simulink model "Model_6DOF"  (R2020b)
settings: Solver=FixedStepAuto  StartTime=0.0  StopTime=Tfin  FixedStep=0.05  RelTol=1e-3
values from neighbouring files (symbols this model uses):
  Ba_0 = [0 0 0 0 0 0]    [ctrl_mode_param.m]
  Bb = 4418825.3321    [load_data.m]
  Bv_0 = [tgt_speed 0 0 0 0 0]    [ctrl_mode_param.m]
  Bx_0 = [0 0 tgt_depth 0 0 0]    [ctrl_mode_param.m]
  check_angle = 10    [ctrl_mode_param.m]
  ctrl_mode = 2    [run.m]
  dX_imposed = 10    [ctrl_mode_param.m]
  Ixx = 5.23e7    (= 52300000)    [load_data.m]
  Ixy = 0    [load_data.m]
  Ixz = 0    [load_data.m]
  Iyy = 1.375e9    (= 1375000000)    [load_data.m]
  Iyz = 0    [load_data.m]
  Izz = 1.367e9    (= 1367000000)    [load_data.m]
  Mb = 4418825.3321    [load_data.m]
  Seastate = 5    [ctrl_mode_param.m]    (also in run.m = 0)
  tgt_depth = -100    [ctrl_mode_param.m]
  tgt_pitch = 0    [ctrl_mode_param.m]
  tgt_speed = -4.72    [ctrl_mode_param.m]
  tgt_sway = 0    [ctrl_mode_param.m]
  tgt_yaw = 0    [ctrl_mode_param.m]
  Xb = 0    [load_data.m]
  Xcg = [32.3114*1.0005364451; 0; 0;]    [load_data.m]
  Xg = 0    [load_data.m]
  Yb = 0    [load_data.m]
  Yg = 0    [load_data.m]
  Zb = 0.4406    [load_data.m]
  Zg = 0    [load_data.m]
undefined symbols (not defined in the file or in its folder): dA_BP1, dA_BP2, dA_Hull, dA_PH, dA_Sail, dA_SProot, dA_X1a, dA_X1b, dA_X2a, dA_X2b, dA_X3a, dA_X3b, dA_X4a, dA_X4b, n_BP1, n_BP2, n_Hull, n_PH, n_Sail, n_SProot, n_X2a, n_X2b, n_X3a, n_X4a, n_X4b, nt_BP1, nt_BP2, nt_Hull, nt_PH, nt_Sail, nt_SProot, nt_X1a, nt_X1b, nt_X2a, nt_X2b, nt_X3a, nt_X3b, nt_X4a, nt_X4b, vt1_BP1, vt1_BP2, vt1_Hull, vt1_PH, vt1_Sail, vt1_SProot, vt1_X1a, vt1_X1b, vt1_X2a, vt1_X2b, vt1_X3a, vt1_X3b, vt1_X4a, vt1_X4b, vt2_BP1, vt2_BP2, vt2_Hull, vt2_PH, vt2_Sail, vt2_SProot, vt2_X1a ... (+21)
libraries: simulink x23
(part 6 of 6)

== matlab function Model_6DOF/HDM/HDM B3/Wave, Virtual Mass and Hydrostatic/Wave Particle Motions/Sectional Wave Particle & Rigid Body Velocities ==
  data: time input; U_ship input; X_earth input; Xce input size=[15 3]; Rs input size=[15 3]; phi_wave input; beta_wave input; Uws output size=[15 3]; L_wave input; A_wave input; k_wave input; w_wave input; Urs output size=[15 3]
function [Uws,Urs] = fcn(time,U_ship,X_earth,Xce,Rs,phi_wave,beta_wave,L_wave,A_wave,k_wave,w_wave)
%Inputs
%Rs      : Position vector of each sectional component in ship system.
%X_earth : Global ship position in the earth coordinate system
%U_ship  : Ship's velocity at CG in the ship coordinate system
%L, A, T, k, w of wave: wave properties for given sea state

%Outputs
%Uws: Sectional wave particle velcity vector in ship coordinate system
%Urs: Sectional rigid body translationl velocity vector in ship coordinate system

phi= X_earth(4); theta= X_earth(5); psi= X_earth(6); % Euler angles
u_s= U_ship(1); v_s=U_ship(2); w_s=U_ship(3); p_s= U_ship(4); q_s=U_ship(5); r_s=U_ship(6);

ni = 15; %length(Xce); %number, and the order of sectional elements

Uws = zeros(15,3); Urs = zeros(15,3);
uweBow=zeros(3,1); uweStern=zeros(3,1); uweBP=zeros(3,1);
ursProbe=zeros(3,1);

uri=zeros(15,1); vri=zeros(15,1); wri=zeros(15,1);
uwi=zeros(15,1); vwi=zeros(15); wwi=zeros(15,1);

Omega_s = [p_s; q_s; r_s;]; %angular velocity of the CG in ship coordinate system
Us_CG   = [u_s; v_s; w_s;]; %Translational velocity of the CG in ship coordinate system

RMat=[cos(theta)*cos(psi) -cos(phi)*sin(psi)+sin(phi)*sin(theta)*cos(psi)  sin(phi)*sin(psi)+cos(phi)*sin(theta)*cos(psi); ...
      cos(theta)*sin(psi)  cos(phi)*cos(psi)+sin(phi)*sin(theta)*sin(psi) -sin(phi)*cos(psi)+cos(phi)*sin(theta)*sin(psi); ...
     -sin(theta)                             sin(phi)*cos(theta)                             cos(phi)*cos(theta)];

%phi_wave  = 0; % wave phase. parameterized
%beta_wave = 0; % wave heading. parameterized

    for i= 1:15
        u_w=-A_wave*w_wave*exp(k_wave*Xce(i,3))*cos(k_wave*Xce(i,1)-w_wave*time+phi_wave)*cos(pi*beta_wave);
        v_w= A_wave*w_wave*exp(k_wave*Xce(i,3))*cos(k_wave*Xce(i,1)-w_wave*time+phi_wave)*sin(pi*beta_wave);
        w_w=-A_wave*w_wave*exp(k_wave*Xce(i,3))*sin(k_wave*Xce(i,1)-w_wave*time+phi_wave);
        
        v1=u_w; v2=v_w; v3=w_w;
        uwi(i,1)=v1; vwi(i,1)=v2; wwi(i,1)=v3;
        
        Uwe = [u_w; v_w; w_w;];
        Uint= inv(RMat)*Uwe;
        Uws(i,:) = Uint(:);  %keep Uws for further use in wave AOA calculation     

        if i==1
            uweBow=Uwe;
        elseif i==10
            uweStern=Uwe;
        elseif i==14
            uweBP=Uwe;
        end
        
    end
    
    %Computation of translational velcity of volumetric center of sections.   
    for i=1:15
        r_i      = [Rs(i,1); Rs(i,2); Rs(i,3)];
        Ur_int   = Us_CG + cross(Omega_s,r_i); %cross(r_i,Omega_s);
        
        v1=Ur_int(1); v2=Ur_int(2); v3=Ur_int(3); 
        uri(i,1)=v1; vri(i,1)=v2; wri(i,1)=v3;
        
        for j=1:3
            Urs(i,j)=Ur_int(j);    
        end
    end

end

== matlab function Model_6DOF/HDM/HDM B3/Wave, Virtual Mass and Hydrostatic/Wave Particle Motions/Hydrostatic Forces and Moments/Subsystem/MATLAB Function3 ==
  data: time input; Xearth input; Fx_total output; vert1 input; vert2 input; vert3 input; dA input; ntri input; normal input; A_wave input; k_wave input; w_wave input; rho input; g input; Fy_total output; Fz_total output; Mx_total output; My_total output; Mz_total output; Zb input
function [Fx_total,Fy_total,Fz_total,Mx_total,My_total,Mz_total]= fcn(time,Xearth,vert1,vert2,vert3,dA,ntri,normal,A_wave,k_wave,w_wave,rho,g,Zb)
x_e=Xearth(1); y_e=Xearth(2); z_e=Xearth(3);
phi=Xearth(4); theta=Xearth(5); psi=Xearth(6);

RMat=[cos(theta)*cos(psi) -cos(phi)*sin(psi)+sin(phi)*sin(theta)*cos(psi)  sin(phi)*sin(psi)+cos(phi)*sin(theta)*cos(psi); ...
      cos(theta)*sin(psi)  cos(phi)*cos(psi)+sin(phi)*sin(theta)*sin(psi) -sin(phi)*cos(psi)+cos(phi)*sin(theta)*sin(psi); ...
     -sin(theta)                             sin(phi)*cos(theta)                             cos(phi)*cos(theta)];  

%position of mid points in earth coordinate;
mp1=zeros(ntri,3);
mp2=zeros(ntri,3);
mp3=zeros(ntri,3);
nA =zeros(ntri,3);

P1=zeros(ntri,1);
P2=zeros(ntri,1);
P3=zeros(ntri,1);

%position vector of mid points from the CG
r1=zeros(ntri,3);
r2=zeros(ntri,3);
r3=zeros(ntri,3);
v1_w=zeros(ntri,3);
v2_w=zeros(ntri,3);
v3_w=zeros(ntri,3);
n_w=zeros(ntri,3);

%Area of triangle, product of area and unit normal, position vector to each mid-point
for i=1:ntri
    %Area of each triangle
    A=[vert2(i,1)-vert1(i,1); vert2(i,2)-vert1(i,2); vert2(i,3)-vert1(i,3);];
    B=[vert3(i,1)-vert1(i,1); vert3(i,2)-vert1(i,2); vert3(i,3)-vert1(i,3);];
    C=[normal(i,1); normal(i,2); normal(i,3);];
        
    %A*n vector calculation
    for j=1:3
        nA(i,j)=dA(i).*C(j);    
    end
    
    %position vector to each mid point of each edge
    for j=1:3
        r1(i,j)=0.5*(vert1(i,j)+vert2(i,j));
        r2(i,j)=0.5*(vert1(i,j)+vert3(i,j));
        r3(i,j)=0.5*(vert2(i,j)+vert3(i,j));
    end
end

%computing mid point location between vertices in earth coordinate
for i=1:ntri
    MP1=RMat*[r1(i,1); r1(i,2); r1(i,3);]+[x_e; y_e; z_e;];
    MP2=RMat*[r2(i,1); r2(i,2); r2(i,3);]+[x_e; y_e; z_e;];
    MP3=RMat*[r3(i,1); r3(i,2); r3(i,3);]+[x_e; y_e; z_e;];
    
    v1i=RMat*[vert1(i,1); vert1(i,2); vert1(i,3);]+[x_e; y_e; z_e;];
    v2i=RMat*[vert2(i,1); vert2(i,2); vert2(i,3);]+[x_e; y_e; z_e;];
    v3i=RMat*[vert3(i,1); vert3(i,2); vert3(i,3);]+[x_e; y_e; z_e;];
   
    for j=1:3
        v1_w(i,j)=v1i(j); v2_w(i,j)=v2i(j); v3_w(i,j)=v3i(j); 
        mp1(i,j)=MP1(j);  mp2(i,j)=MP2(j);  mp3(i,j)=MP3(j);
    end
end

for i=1:ntri
    A=[v2_w(i,1)-v1_w(i,1); v2_w(i,2)-v1_w(i,2); v2_w(i,3)-v1_w(i,3);];
    B=[v3_w(i,1)-v1_w(i,1); v3_w(i,2)-v1_w(i,2); v3_w(i,3)-v1_w(i,3);];
    n=cross(A,B)/norm(cross(A,B));
    dA(i,1)=0.5*norm(cross(A,B));
    n_w(i,1)=n(1); n_w(i,2)=n(2); n_w(i,3)=n(3);
end



%computing forces and moments for each triangle
Fx_total=0; Fy_total=0; Fz_total=0;
Mx_total=0; My_total=0; Mz_total=0;

for i=1:ntri
    p1=-rho*g*(mp1(i,3)-A_wave*exp(k_wave.*mp1(i,3)).*sin(k_wave*mp1(i,1)-w_wave.*time));
    p2=-rho*g*(mp2(i,3)-A_wave*exp(k_wave.*mp2(i,3)).*sin(k_wave*mp2(i,1)-w_wave.*time));
    p3=-rho*g*(mp3(i,3)-A_wave*exp(k_wave.*mp3(i,3)).*sin(k_wave*mp3(i,1)-w_wave.*time));
    
    dFx=-nA(i,1)*(p1+p2+p3)./3;
    dFy=-nA(i,2)*(p1+p2+p3)./3;
    dFz=-nA(i,3)*(p1+p2+p3)./3;
    
    dP =-p1.*[r1(i,1); r1(i,2); r1(i,3)-Zb;]...
        -p2.*[r2(i,1); r2(i,2); r2(i,3)-Zb;]...
        -p3.*[r3(i,1); r3(i,2); r3(i,3)-Zb;];
    N =[nA(i,1); nA(i,2); nA(i,3);];
    dM=cross(dP,N);
    Fx_total=Fx_total+dFx;
    Fy_total=Fy_total+dFy;
    Fz_total=Fz_total+dFz;
    Mx_total=Mx_total+dM(1)/3;
    My_total=My_total+dM(2)/3;
    Mz_total=Mz_total+dM(3)/3;
end
end

== matlab function Model_6DOF/HDM/HDM B3/Wave, Virtual Mass and Hydrostatic/Wave Particle Motions/Hydrostatic Forces and Moments/Subsystem/MATLAB Function4 ==
  data: time input; Xearth input; Fx_total output; vert1 input; vert2 input; vert3 input; dA input; ntri input; normal input; A_wave input; k_wave input; w_wave input; rho input; g input; Fy_total output; Fz_total output; Mx_total output; My_total output; Mz_total output; Zb input
function [Fx_total,Fy_total,Fz_total,Mx_total,My_total,Mz_total]= fcn(time,Xearth,vert1,vert2,vert3,dA,ntri,normal,A_wave,k_wave,w_wave,rho,g,Zb)
x_e=Xearth(1); y_e=Xearth(2); z_e=Xearth(3);
phi=Xearth(4); theta=Xearth(5); psi=Xearth(6);

RMat=[cos(theta)*cos(psi) -cos(phi)*sin(psi)+sin(phi)*sin(theta)*cos(psi)  sin(phi)*sin(psi)+cos(phi)*sin(theta)*cos(psi); ...
      cos(theta)*sin(psi)  cos(phi)*cos(psi)+sin(phi)*sin(theta)*sin(psi) -sin(phi)*cos(psi)+cos(phi)*sin(theta)*sin(psi); ...
     -sin(theta)                             sin(phi)*cos(theta)                             cos(phi)*cos(theta)];  

%position of mid points in earth coordinate;
mp1=zeros(ntri,3);
mp2=zeros(ntri,3);
mp3=zeros(ntri,3);
nA =zeros(ntri,3);

P1=zeros(ntri,1);
P2=zeros(ntri,1);
P3=zeros(ntri,1);

%position vector of mid points from the CG
r1=zeros(ntri,3);
r2=zeros(ntri,3);
r3=zeros(ntri,3);
v1_w=zeros(ntri,3);
v2_w=zeros(ntri,3);
v3_w=zeros(ntri,3);
n_w=zeros(ntri,3);

%Area of triangle, product of area and unit normal, position vector to each mid-point
for i=1:ntri
    %Area of each triangle
    A=[vert2(i,1)-vert1(i,1); vert2(i,2)-vert1(i,2); vert2(i,3)-vert1(i,3);];
    B=[vert3(i,1)-vert1(i,1); vert3(i,2)-vert1(i,2); vert3(i,3)-vert1(i,3);];
    C=[normal(i,1); normal(i,2); normal(i,3);];
        
    %A*n vector calculation
    for j=1:3
        nA(i,j)=dA(i).*C(j);    
    end
    
    %position vector to each mid point of each edge
    for j=1:3
        r1(i,j)=0.5*(vert1(i,j)+vert2(i,j));
        r2(i,j)=0.5*(vert1(i,j)+vert3(i,j));
        r3(i,j)=0.5*(vert2(i,j)+vert3(i,j));
    end
end

%computing mid point location between vertices in earth coordinate
for i=1:ntri
    MP1=RMat*[r1(i,1); r1(i,2); r1(i,3);]+[x_e; y_e; z_e;];
    MP2=RMat*[r2(i,1); r2(i,2); r2(i,3);]+[x_e; y_e; z_e;];
    MP3=RMat*[r3(i,1); r3(i,2); r3(i,3);]+[x_e; y_e; z_e;];
    
    v1i=RMat*[vert1(i,1); vert1(i,2); vert1(i,3);]+[x_e; y_e; z_e;];
    v2i=RMat*[vert2(i,1); vert2(i,2); vert2(i,3);]+[x_e; y_e; z_e;];
    v3i=RMat*[vert3(i,1); vert3(i,2); vert3(i,3);]+[x_e; y_e; z_e;];
   
    for j=1:3
        v1_w(i,j)=v1i(j); v2_w(i,j)=v2i(j); v3_w(i,j)=v3i(j); 
        mp1(i,j)=MP1(j);  mp2(i,j)=MP2(j);  mp3(i,j)=MP3(j);
    end
end

for i=1:ntri
    A=[v2_w(i,1)-v1_w(i,1); v2_w(i,2)-v1_w(i,2); v2_w(i,3)-v1_w(i,3);];
    B=[v3_w(i,1)-v1_w(i,1); v3_w(i,2)-v1_w(i,2); v3_w(i,3)-v1_w(i,3);];
    n=cross(A,B)/norm(cross(A,B));
    dA(i,1)=0.5*norm(cross(A,B));
    n_w(i,1)=n(1); n_w(i,2)=n(2); n_w(i,3)=n(3);
end


%computing forces and moments for each triangle
Fx_total=0; Fy_total=0; Fz_total=0;
Mx_total=0; My_total=0; Mz_total=0;

for i=1:ntri
    p1=-rho*g*(mp1(i,3)-A_wave*exp(k_wave.*mp1(i,3)).*sin(k_wave*mp1(i,1)-w_wave.*time));
    p2=-rho*g*(mp2(i,3)-A_wave*exp(k_wave.*mp2(i,3)).*sin(k_wave*mp2(i,1)-w_wave.*time));
    p3=-rho*g*(mp3(i,3)-A_wave*exp(k_wave.*mp3(i,3)).*sin(k_wave*mp3(i,1)-w_wave.*time));
    
    dFx=-nA(i,1)*(p1+p2+p3)./3;
    dFy=-nA(i,2)*(p1+p2+p3)./3;
    dFz=-nA(i,3)*(p1+p2+p3)./3;
    
    dP =-p1.*[r1(i,1); r1(i,2); r1(i,3)-Zb;]...
        -p2.*[r2(i,1); r2(i,2); r2(i,3)-Zb;]...
        -p3.*[r3(i,1); r3(i,2); r3(i,3)-Zb;];
    N =[nA(i,1); nA(i,2); nA(i,3);];
    dM=cross(dP,N);
    Fx_total=Fx_total+dFx;
    Fy_total=Fy_total+dFy;
    Fz_total=Fz_total+dFz;
    Mx_total=Mx_total+dM(1)/3;
    My_total=My_total+dM(2)/3;
    Mz_total=Mz_total+dM(3)/3;
end
end

== matlab function Model_6DOF/HDM/HDM B3/Wave, Virtual Mass and Hydrostatic/Wave Particle Motions/Wave Properties ==
  data: SeaState input; L_wave output; A_wave output; k_wave output; w_wave output
function [L_wave,A_wave,k_wave,w_wave] = fcn(SeaState)

   if SeaState==2;
       L_wave= 87.8; A_wave= 0.15;
   elseif SeaState==3;
       L_wave= 87.8; A_wave= 0.44;
   elseif SeaState==4;
       L_wave= 120.9; A_wave= 0.94;
   elseif SeaState==5;
       L_wave= 140.9; A_wave= 1.625;
   elseif SeaState==6;
       L_wave=240.1; A_wave=2.5;
   elseif SeaState==7;
       L_wave= 351.3; A_wave= 3.750;
   else
       L_wave= 0; A_wave=0;
   end
   
   if(L_wave==0)
       k_wave=0;
   else
       k_wave=2*pi/L_wave;
   end
   
   w_wave=sqrt(9.81*k_wave);
   
end

== matlab function Model_6DOF/HDM/HDM B3/Wave, Virtual Mass and Hydrostatic/Wave Particle Motions/Wave particle velocity at hull CG ==
  data: time input; X_earth input; uwsCG output; dLCG input; L_wave input; phi_wave input; beta_wave input; A_wave input; k_wave input; w_wave input
function uwsCG  = fcn(time,X_earth,dLCG,L_wave,phi_wave,beta_wave,A_wave,k_wave,w_wave)
 
    Xs=[X_earth(1); X_earth(2); X_earth(3);];
    phi= X_earth(4); theta= X_earth(5); psi= X_earth(6); % Euler angles
    
    RMat=[cos(theta)*cos(psi) -cos(phi)*sin(psi)+sin(phi)*sin(theta)*cos(psi)  sin(phi)*sin(psi)+cos(phi)*sin(theta)*cos(psi); ...
          cos(theta)*sin(psi)  cos(phi)*cos(psi)+sin(phi)*sin(theta)*sin(psi) -sin(phi)*cos(psi)+cos(phi)*sin(theta)*sin(psi); ...
        -sin(theta)                             sin(phi)*cos(theta)                             cos(phi)*cos(theta)];  

    u_w=-A_wave*w_wave*exp(k_wave*Xs(3))*cos(k_wave*Xs(1)-w_wave*time+phi_wave)*cos(pi*beta_wave);
    v_w= A_wave*w_wave*exp(k_wave*Xs(3))*cos(k_wave*Xs(1)-w_wave*time+phi_wave)*sin(pi*beta_wave);
    w_w=-A_wave*w_wave*exp(k_wave*Xs(3))*sin(k_wave*Xs(1)-w_wave*time+phi_wave);
    
    uweCG = [u_w; v_w; w_w;];
    uwsCG = inv(RMat)*uweCG;
    
end

== matlab function Model_6DOF/HDM/HDM B3/X/Fx ==
  data: Bx input; Bv input; Ba input; CXqq input; CXuvwV input; CXuvwH input; Umag input; dLCG input; dmass input; UeSP input; XdXi input; X output; Tprop input; Mb parameter; Bb parameter; Xvm input; Xapp output; Xhull output; Tout output; X_Hyd output; XdX output; BFX input; Xstat output
function [X,Xapp,Xhull,Tout,X_Hyd,XdX,Xstat]   = fcn(Bx,Bv,Ba,CXqq,CXuvwV,CXuvwH,Umag,dLCG,dmass,UeSP,XdXi,Tprop,Mb,Bb,Xvm,BFX)
%Bx,Bv,Ba are the body motion position, velocity, acceleration in ship coordinate
%Wv,Wa are the wave particle velocity, acceleration in ship coordinate

u=Bv(1); v=Bv(2); w=Bv(3); p=Bv(4); q=Bv(5); r=Bv(6);
x=Bx(1); y=Bx(2); z=Bx(3); phi=Bx(4); theta=Bx(5); psi=Bx(6);
a1=Ba(1); a2=Ba(2); a3=Ba(3); a4=Ba(4); a5=Ba(5); a6=Ba(6); 

%Xwq=1025*70.2^3*CXwq
%Twq=0.5*1025*70.2^3*CTwq
%Xstat=BFX-(Mb+dmass)*9.81*sin(Bx(5));%-((Mb+dmass)-Bb)*9.81*sin(Bx(5));

Xqq=0.5*1025*70.2^4*q^2*CXqq;
Xwq=1025*70.2^3*(-3.3124286E-03*w*q)
Xvr=1025*70.2^3*(-3.3124286E-03*v*r)*0
Twq=0.5*1025*70.2^3*(3.6594E-03*w*q)
Tvr=0.5*1025*70.2^3*(3.6594E-03*v*r)*0

dXiuq=(4.4603E-03*(u*q)^2-7.3687E-06*(u*q))


XX1=0.5*1025*70.2^2*(XdXi(1)+dXiuq)*UeSP(1)^2
XX2=0.5*1025*70.2^2*(XdXi(2)+dXiuq)*UeSP(2)^2
XX3=0.5*1025*70.2^2*(XdXi(3)+dXiuq)*UeSP(3)^2
XX4=0.5*1025*70.2^2*(XdXi(4)+dXiuq)*UeSP(4)^2
XXB=0.5*1025*(70.2^2*XdXi(5)*UeSP(5)^2)

XdX=[XX1; XX2; XX3; XX4; XXB;]

Xapp=XX1+XX2+XX3+XX4+XXB;
Xuvw=-0.5*1025*70.2^2*(CXuvwV+CXuvwH)*Umag^2*u/abs(u);
Xstat=BFX+(Mb+dmass)*9.81*sin(Bx(5))
Xhull=Xqq+Xuvw+Xwq+Xvr;
Tout=Tprop+Twq+Tvr;
X_Hyd=Xapp+Xhull+Xstat-Tout;
X=Xapp+Xhull+Xstat-Tout+Xvm;

== matlab function Model_6DOF/HDM/HDM B3/Wave, Virtual Mass and Hydrostatic/Wave Particle Motions/Hydrostatic Forces and Moments/Subsystem/MATLAB Function5 ==
  data: time input; Xearth input; Fx_total output; vert1 input; vert2 input; vert3 input; dA input; ntri input; normal input; A_wave input; k_wave input; w_wave input; rho input; g input; Fy_total output; Fz_total output; Mx_total output; My_total output; Mz_total output; Zb input
function [Fx_total,Fy_total,Fz_total,Mx_total,My_total,Mz_total]= fcn(time,Xearth,vert1,vert2,vert3,dA,ntri,normal,A_wave,k_wave,w_wave,rho,g,Zb)
x_e=Xearth(1); y_e=Xearth(2); z_e=Xearth(3);
phi=Xearth(4); theta=Xearth(5); psi=Xearth(6);

RMat=[cos(theta)*cos(psi) -cos(phi)*sin(psi)+sin(phi)*sin(theta)*cos(psi)  sin(phi)*sin(psi)+cos(phi)*sin(theta)*cos(psi); ...
      cos(theta)*sin(psi)  cos(phi)*cos(psi)+sin(phi)*sin(theta)*sin(psi) -sin(phi)*cos(psi)+cos(phi)*sin(theta)*sin(psi); ...
     -sin(theta)                             sin(phi)*cos(theta)                             cos(phi)*cos(theta)];  

%position of mid points in earth coordinate;
mp1=zeros(ntri,3);
mp2=zeros(ntri,3);
mp3=zeros(ntri,3);
nA =zeros(ntri,3);

P1=zeros(ntri,1);
P2=zeros(ntri,1);
P3=zeros(ntri,1);

%position vector of mid points from the CG
r1=zeros(ntri,3);
r2=zeros(ntri,3);
r3=zeros(ntri,3);
v1_w=zeros(ntri,3);
v2_w=zeros(ntri,3);
v3_w=zeros(ntri,3);
n_w=zeros(ntri,3);

%Area of triangle, product of area and unit normal, position vector to each mid-point
for i=1:ntri
    %Area of each triangle
    A=[vert2(i,1)-vert1(i,1); vert2(i,2)-vert1(i,2); vert2(i,3)-vert1(i,3);];
    B=[vert3(i,1)-vert1(i,1); vert3(i,2)-vert1(i,2); vert3(i,3)-vert1(i,3);];
    C=[normal(i,1); normal(i,2); normal(i,3);];
        
    %A*n vector calculation
    for j=1:3
        nA(i,j)=dA(i).*C(j);    
    end
    
    %position vector to each mid point of each edge
    for j=1:3
        r1(i,j)=0.5*(vert1(i,j)+vert2(i,j));
        r2(i,j)=0.5*(vert1(i,j)+vert3(i,j));
        r3(i,j)=0.5*(vert2(i,j)+vert3(i,j));
    end
end

%computing mid point location between vertices in earth coordinate
for i=1:ntri
    MP1=RMat*[r1(i,1); r1(i,2); r1(i,3);]+[x_e; y_e; z_e;];
    MP2=RMat*[r2(i,1); r2(i,2); r2(i,3);]+[x_e; y_e; z_e;];
    MP3=RMat*[r3(i,1); r3(i,2); r3(i,3);]+[x_e; y_e; z_e;];
    
    v1i=RMat*[vert1(i,1); vert1(i,2); vert1(i,3);]+[x_e; y_e; z_e;];
    v2i=RMat*[vert2(i,1); vert2(i,2); vert2(i,3);]+[x_e; y_e; z_e;];
    v3i=RMat*[vert3(i,1); vert3(i,2); vert3(i,3);]+[x_e; y_e; z_e;];
   
    for j=1:3
        v1_w(i,j)=v1i(j); v2_w(i,j)=v2i(j); v3_w(i,j)=v3i(j); 
        mp1(i,j)=MP1(j);  mp2(i,j)=MP2(j);  mp3(i,j)=MP3(j);
    end
end

for i=1:ntri
    A=[v2_w(i,1)-v1_w(i,1); v2_w(i,2)-v1_w(i,2); v2_w(i,3)-v1_w(i,3);];
    B=[v3_w(i,1)-v1_w(i,1); v3_w(i,2)-v1_w(i,2); v3_w(i,3)-v1_w(i,3);];
    n=cross(A,B)/norm(cross(A,B));
    dA(i,1)=0.5*norm(cross(A,B));
    n_w(i,1)=n(1); n_w(i,2)=n(2); n_w(i,3)=n(3);
end



%computing forces and moments for each triangle
Fx_total=0; Fy_total=0; Fz_total=0;
Mx_total=0; My_total=0; Mz_total=0;

for i=1:ntri
    p1=-rho*g*(mp1(i,3)-A_wave*exp(k_wave.*mp1(i,3)).*sin(k_wave*mp1(i,1)-w_wave.*time));
    p2=-rho*g*(mp2(i,3)-A_wave*exp(k_wave.*mp2(i,3)).*sin(k_wave*mp2(i,1)-w_wave.*time));
    p3=-rho*g*(mp3(i,3)-A_wave*exp(k_wave.*mp3(i,3)).*sin(k_wave*mp3(i,1)-w_wave.*time));
    
    dFx=-nA(i,1)*(p1+p2+p3)./3;
    dFy=-nA(i,2)*(p1+p2+p3)./3;
    dFz=-nA(i,3)*(p1+p2+p3)./3;
    
    dP =-p1.*[r1(i,1); r1(i,2); r1(i,3)-Zb;]...
        -p2.*[r2(i,1); r2(i,2); r2(i,3)-Zb;]...
        -p3.*[r3(i,1); r3(i,2); r3(i,3)-Zb;];
    N =[nA(i,1); nA(i,2); nA(i,3);];
    dM=cross(dP,N);
    Fx_total=Fx_total+dFx;
    Fy_total=Fy_total+dFy;
    Fz_total=Fz_total+dFz;
    Mx_total=Mx_total+dM(1)/3;
    My_total=My_total+dM(2)/3;
    Mz_total=Mz_total+dM(3)/3;
end
end

== matlab function Model_6DOF/HDM/HDM B3/Thrust & Torque/Tprop ==
  data: speed input; Td input; Tprop output; n_0 input; Qprop output
function [Tprop,Qprop]   = fcn(speed,Td,n_0)
J=speed/(n_0*5);
Kt=-0.0923*J^2-0.3652*J+0.4786;
Kq=-2.1064E-02*J^2 - 3.2470E-02*J + 6.3982E-02;
Tprop=Kt*(1-Td)*(1025*n_0^2*5^4);
Qprop=Kq*1025*n_0^2*5^5

== matlab function Model_6DOF/HDM/HDM B3/Y/Fy ==
  data: Bx input; Bv input; Ba input; CYr input; CYvr input; CYrr input; CYuvw input; Umag input; UeX input; dLCG input; dmass input; CYdXi input; Mb parameter; Bb parameter; Fy output; FYApp output; FYhull output; FY_hyd output; FYprop output; Yvm input; FYAppAll output; BFY input; FYHullVM output
 function [Fy,FYApp,FYhull,FY_hyd,FYprop,FYAppAll,FYHullVM]  = fcn(Bx,Bv,Ba,CYr,CYvr,CYrr,CYuvw,Umag,UeX,dLCG,dmass,CYdXi,Mb,Bb,Yvm,BFY)
%Bx,Bv,Ba are the body motion position, velocity, acceleration in ship coordinate
%Wv,Wa are the wave particle velocity, acceleration in ship coordinate
 
u=Bv(1); v=Bv(2); w=Bv(3); p=Bv(4); q=Bv(5); r=Bv(6);
x=Bx(1); y=Bx(2); z=Bx(3); phi=Bx(4); theta=Bx(5); psi=Bx(6);
a1=Ba(1); a2=Ba(2); a3=Ba(3); a4=Ba(4); a5=Ba(5); a6=Ba(6); 

FYuvw=0.5*1025*70.2^2*CYuvw*Umag^2

FYx1=1025*70.2^2*CYdXi(1)*UeX(1)^2
FYx2=1025*70.2^2*CYdXi(2)*UeX(2)^2
FYx3=1025*70.2^2*CYdXi(3)*UeX(3)^2
FYx4=1025*70.2^2*CYdXi(4)*UeX(4)^2

FYrr=0.5*1025*70.2^4*CYrr*q*abs(q)*0
FYr =-1025*70.2^2*(0.9*8.2086E-03*u*r)*u^2*2

FYAppAll=[FYx1; FYx2 ;FYx3; FYx4;]

%FYr =0.5*1025*70.2^3*CYr*u^2*2
FYvr=0.5*1025*70.2^3*CYvr*u^2*0
FYprop=0;
FYhull=FYuvw+FYr+FYvr+FYrr
FYHullVM=FYhull+Yvm
FYApp=FYx1+FYx2+FYx3+FYx4
FYStat=(Mb+dmass)*9.81*cos(theta)*sin(phi)-BFY %((Mb+dmass)-Bb)*9.81*cos(theta)*sin(phi)
FY_hyd=FYApp+FYStat+FYhull+FYprop
Fy=FYApp+FYStat+FYhull+Yvm+FYprop
 end

== matlab function Model_6DOF/HDM/HDM B3/Z/Fz ==
  data: Bx input; Bv input; Ba input; Zqq input; Zuq input; Zwq input; Zuvw_a input; Zuvw_b input; CZProp input; Umag input; UeSP input; dLCG input; dmass input; ZdXi input; Mb parameter; Bb parameter; Fz output; Zvm input; FZApp output; FZHull output; FZProp output; FZ_Hyd output; FZApp_All output; BFZ input
 function [Fz,FZApp,FZHull,FZProp,FZ_Hyd,FZApp_All]  = fcn(Bx,Bv,Ba,Zqq,Zuq,Zwq,Zuvw_a,Zuvw_b,CZProp,Umag,UeSP,dLCG,dmass,ZdXi,Mb,Bb,Zvm,BFZ)
%Bx,Bv,Ba are the body motion position, velocity, acceleration in ship coordinate
%Wv,Wa are the wave particle velocity, acceleration in ship coordinate
 
u=Bv(1); v=Bv(2); w=Bv(3); p=Bv(4); q=Bv(5); r=Bv(6);
x=Bx(1); y=Bx(2); z=Bx(3); phi=Bx(4); theta=Bx(5); psi=Bx(6);
a1=Ba(1); a2=Ba(2); a3=Ba(3); a4=Ba(4); a5=Ba(5); a6=Ba(6); 

FZProp=0.5*1025*70.2^3*CZProp;

FZx1=0.5*1025*70.2^2*ZdXi(1)*UeSP(1)^2;
FZx2=0.5*1025*70.2^2*ZdXi(2)*UeSP(2)^2;
FZx3=0.5*1025*70.2^2*ZdXi(3)*UeSP(3)^2;
FZx4=0.5*1025*70.2^2*ZdXi(4)*UeSP(4)^2;
FZxb=0.5*1025*70.2^2*ZdXi(5)*UeSP(5)^2;

FZqq=0.5*1025*70.2^4*Zqq*q^2*5.1444^2;
FZuq=(-0.01066*u*q)*0.5*70.2^3*1025*0.6;
FZur=(1.5483E-03*u*r)*70.2^2*1025*5.1444^2;
FZwq=0.5*1025*70.2^3*Zwq*w*abs(q);

FZApp_All=[FZx1; FZx2; FZx3; FZx4; FZxb;];

FZApp=(FZx1+FZx2+FZx3+FZx4+FZxb);
FZuvw=0.5*1025*70.2^2*(Zuvw_a+Zuvw_b*2)*Umag^2;
FZStat=BFZ-((Mb+dmass))*9.81*cos(theta);
FZHull=FZuvw+FZqq+FZuq+FZur;
FZ_Hyd=FZApp+FZStat+FZHull+FZProp;
Fz=FZApp+FZStat+FZHull+FZProp+Zvm;
end

== matlab function Model_6DOF/HDM/HDM B3/Z/Linearized Zuvw ==
  data: x input; y output
function y = fcn(x)
y=2.5079E-04*1*x + 1.9855E-05
end
